simulink model "AerialPlatformTotal_Modified"  (R2023a)
settings: Solver=VariableStepAuto  StartTime=0.0  StopTime=10.0  RelTol=1e-3
model workspace: external: MATLAB File E:\ML & Control\1- Be A Part Of Science Community (Stick Your Head Out)\AerialInspection-IndustrialStacks\MATLAB\Simulation\AerialPlatformTotal_DataFile.m (data not in the file)
values from neighbouring files (symbols this model uses):
  X = T*[x0;y0]    [line2circle.m]
undefined symbols (not defined in the file or in its folder): smiData, Y, Z
libraries: sm_lib x394, nesl_utility x20
(part 1 of 8)
settings Model: Creator=mojtaba  LastModifiedBy=mojtaba

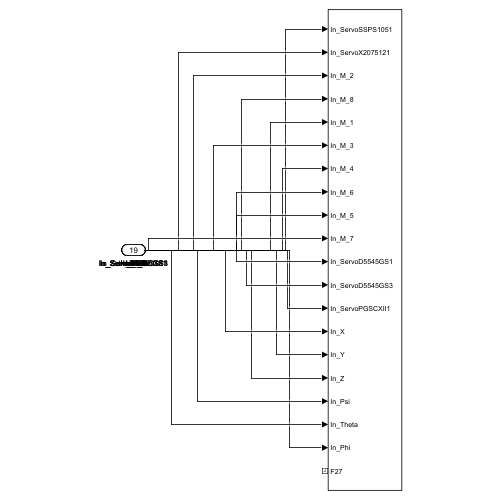
[thumbnail: Simulink's stored preview of the top-level diagram]
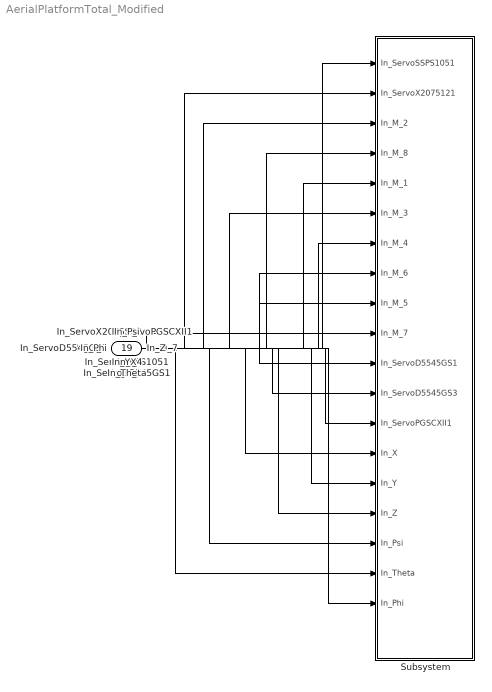
== system AerialPlatformTotal_Modified ==
  In_ServoSSPS1051 : Inport
  In_ServoX2075121 : Inport  Port=2
  In_M_2 : Inport  Port=3
  In_M_8 : Inport  Port=4
  In_M_1 : Inport  Port=5
  In_M_3 : Inport  Port=6
  In_M_4 : Inport  Port=7
  In_M_6 : Inport  Port=8
  In_M_5 : Inport  Port=9
  In_M_7 : Inport  Port=10
  In_ServoD5545GS1 : Inport  Port=11
  In_ServoD5545GS3 : Inport  Port=12
  In_ServoPGSCXII1 : Inport  Port=13
  In_X : Inport  Port=14
  In_Y : Inport  Port=15
  In_Z : Inport  Port=16
  In_Psi : Inport  Port=17
  In_Theta : Inport  Port=18
  In_Phi : Inport  Port=19
  Subsystem : Subsystem
  wires:
  In_Phi/1 -> Subsystem/19(In_Phi)
  In_M_6/1 -> Subsystem/8(In_M_6)
  In_ServoSSPS1051/1 -> Subsystem/1(In_ServoSSPS1051)
  In_ServoX2075121/1 -> Subsystem/2(In_ServoX2075121)
  In_M_2/1 -> Subsystem/3(In_M_2)
  In_M_8/1 -> Subsystem/4(In_M_8)
  In_M_1/1 -> Subsystem/5(In_M_1)
  In_M_3/1 -> Subsystem/6(In_M_3)
  In_M_4/1 -> Subsystem/7(In_M_4)
  In_M_5/1 -> Subsystem/9(In_M_5)
  In_M_7/1 -> Subsystem/10(In_M_7)
  In_ServoD5545GS1/1 -> Subsystem/11(In_ServoD5545GS1)
  In_ServoD5545GS3/1 -> Subsystem/12(In_ServoD5545GS3)
  In_ServoPGSCXII1/1 -> Subsystem/13(In_ServoPGSCXII1)
  In_X/1 -> Subsystem/14(In_X)
  In_Y/1 -> Subsystem/15(In_Y)
  In_Z/1 -> Subsystem/16(In_Z)
  In_Psi/1 -> Subsystem/17(In_Psi)
  In_Theta/1 -> Subsystem/18(In_Theta)
